simulink model "xygraph_demo"  (Simulink 6.3)
settings: Solver=ode45  StartTime=0.0  StopTime=10.0  RelTol=1e-3
libraries: simulink x2
settings Model: LastModifiedBy=Ms1

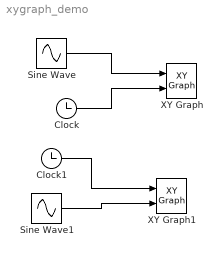
== system xygraph_demo ==
  Clock : Clock
      settings: Decimation=10
  Clock1 : Clock
      settings: Decimation=10
  Sine Wave : Sin  Amplitude=2  Bias=2  Frequency=2  SampleTime=0
  Sine Wave1 : Sin  Amplitude=2  Bias=2  Frequency=2  SampleTime=0
  XY Graph : simulink/Sinks/XY Graph  xmin=0  xmax=5  ymin=0  ymax=5  st=-1
  XY Graph1 : simulink/Sinks/XY Graph  xmin=0  xmax=5  ymin=0  ymax=5  st=-1
  wires:
  Clock/1 -> XY Graph/2
  Sine Wave/1 -> XY Graph/1
  Sine Wave1/1 -> XY Graph1/2
  Clock1/1 -> XY Graph1/1
